simulink model "combinedfb"  (R2016a)
settings: Solver=VariableStepAuto  StartTime=0.0  StopTime=1000  RelTol=1e-3
libraries: simulink x1
settings Model: Creator=sid_1  LastModifiedBy=sid_1

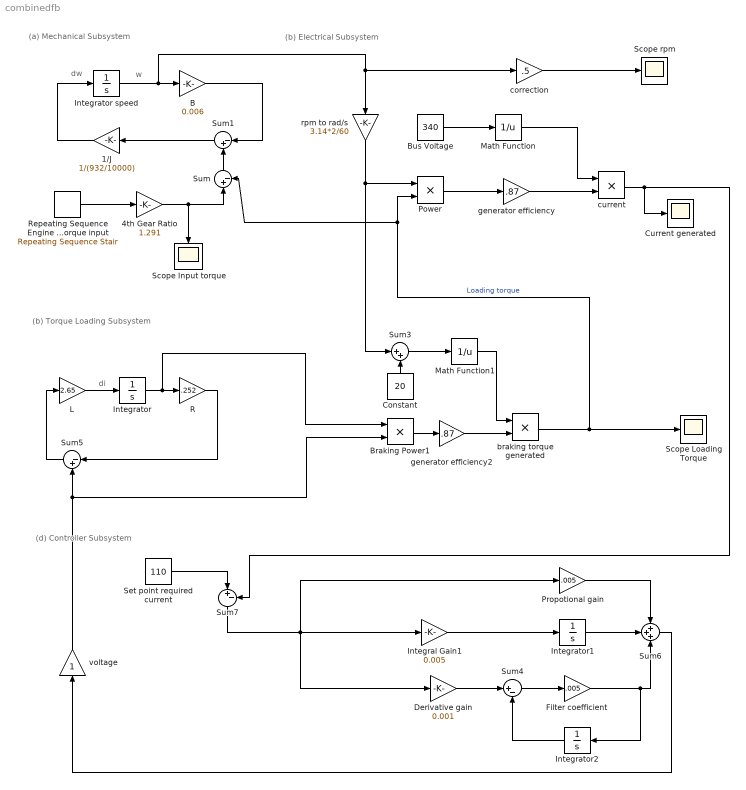
== system combinedfb ==
  note: (b) Electrical Subsystem
  note: (d) Controller Subsystem
  note: (b) Torque Loading Subsystem
  note: (a) Mechanical Subsystem
  note: dw
  note: w
  note: di
  1/J : Gain  Gain=1/(932/10000)
  4th Gear Ratio : Gain  Gain=1.291
  B : Gain  Gain=0.006
  Braking Power1 : Product
  "Bus Voltage " : Constant  Value=340
  Constant : Constant  Value=20
  Current generated : Scope
  Derivative gain : Gain  Gain=0.001
  Filter coefficient : Gain  Gain=.005
  Integral Gain1 : Gain  Gain=0.005
  Integrator : Integrator
  Integrator speed : Integrator
  Integrator1 : Integrator
  Integrator2 : Integrator
  "L " : Gain  Gain=2.65
  Math Function : Math  Operator=reciprocal  SaturateOnIntegerOverflow=on
  Math Function1 : Math  Operator=reciprocal  SaturateOnIntegerOverflow=on
  Power : Product
  Propotional gain : Gain  Gain=.005
  R : Gain  Gain=.252
  Repeating Sequence Engine Torque input : simulink/Sources/Repeating Sequence Stair  OutValues=[1:.45:77 77 77 77 77 77 77 77 77 77 77 77 77 77 77 77 77 77 77 77 77 77 77 77 77 77 77 77 77 77 77 77 77 77 77 77 77 77 77 77 77 77 77 77 77 77 77 77 77 77 77 77 77 77 77 77 77 77 77 77 77 77 77 77 77 77 77 77 77 77 77 77 77 77 77 77 77 77 77 77 77 77 77 77 77 77 77 77 77 77 77 77 77 77 77 77 77 77 77 77 77 77 77 77 77 77 77 77 77 77 77 77 77 77 77 77 77 77 77 77 77 77 77 77 77 77 77 77 77 77 77 77 77 77 77 77 77 77 77 77 77 77 77 77 77 77 77 77 77 77 77 77 77 77 77 77 77 77 77 77 77 77 77 77 77 77 77 77 77 77 77 77 77 77 77 77 77 77 77 77 77 77 77 77 77 77 77 77 77 77 77 77 77 77 77 77 77 77 77 77 77 77 77 77 77 77 77 77 77 77 77 77 77 77 77 77 77 77 77 77 77 77 77 77 77 77 77 77 77 77 77 77 77 77 77 77 77 77 77 77 77 77 77 77 77 77 77 77 77 77 77 77 77 77 77 77 77 77 77 77 77 77 77 77 77 77 77 77 77 77 77 77 77 77 77 77 77 77 77 77 77 77 77 77 77 77 77 77 77 77 77 77 77 77 77 77 77 77 77 77 77 77 77 77 77 77 77 77 77 77 77 77 77 77 77 77 77 77 77 77 77 77 77 77 77 77 77 77 77 77 77 77 77 77 77 77 77 77 77 77 77 77 77 77 77 77 77 77 77 77 77 77 77 77 77 77 77 77 77 77 77 77 77 77 77 77 77 77 77 77 77 77 77 77 77 77 77 77 77 77 77 77 77 77 77 77 77 77 77 77 77 77 77 77 77 77 77 77 77 77 77 77 77 77 77 77 77 77 77 77 77 77 77 77 77 77 77 77 77 77 77 77 77 77 77 77 77 77 77 77 77 77 77 77 77 77 77 77 77 77 77 77 77 77 77 77 77 77 77 77 77 77 77 77 77 77 77 77 77 77 77 77 77 77 77 77 77 77 77 77 77 77 77 77 77 77 77 77 77 77 77 77 77 77 77 77 77 77 77 77 77 77 77 77 77 77 77 77 77 77 77 77 77 77 77 77 77 77 77 77 77 77 77 77 77 77 77 77 77 77 77 77 77 77 77 77 77 77 77 77 77 77 77 77 77 77 77 77 77 77 77 77 77 77 77 77 77 77 77 77 77 77 77 77 77 77 77 77 77 77 77 77 77 77 77 77 77 77 77 77 77 77 77 77 77 77 77 77 77 77 77 77 77 77 77 77 77 77 77 77 77 77 77 77 77 77 77 77 77 77 77 77 77 77 77 77 77 77 77 77 77 77 77 77 77 77 77 77 77 77 77 77 77 77 77 77 77 77 77 77 77 77 77 77 77 77 77 77 77 77 77 77 77 77 77 77 77 77 77 77 77 77 77 77 77 77 77 77 77 77 77 77 77 77 77 77 77 77 77 77 77 77 77 77 77 77 77 77 77 77 77 77 77 77 77 77 77 77 77 77 77 77 77 77 77 77 77 77 77 77 77 77 77 77 77 77 77 77 77 77 77 77 77 77 77 77 77 77 77 77 77 77 77 77 77 77 77 77 77 77 77 77 77 77 77 77 77 77 77 77 77 77 77 77 77 77 77 77 77 77 77 77 77 77 77 77 77 77 77 77 77 77 77 77 77 77 77 77 77 77 77 77 77 77 77 77 77 77 77 77 77 77 77 77 77 77 77 77 77 77 77 77 77 77 77 77 77 77 77 77 77 77 77 77 77 77 77 77 77 77 77 77 77 77 77 77 77 77 77 77 77 77 77 77 77 77 77 77 77 77 77 77 77 77 77 77 77 77 77 77 77 77 77 77 77 77 77 77 77 77 77 77 77 77 77 77 77 77 77 77 77 77 77 77 77 77 77 77 77 77 77 77 77 77 77 77 77 77 77 77 77 77 77 77 77 77 77 77 77 77 77 77 77 77 77 77]  tsamp=1  OutMin=[]  OutMax=[]  OutDataTypeStr=single  OutputDataTypeScalingMode=single  OutDataType=fixdt(0,8)  ConRadixGroup=Best Precision: Vector-wise  OutScaling=2^-12
  Scope Loading Torque : Scope
  Scope rpm : Scope
  Scope Input torque : Scope
  "Set point required current " : Constant  Value=110
  Sum : Sum  Inputs=|+-
  Sum1 : Sum  Inputs=|-+
  Sum3 : Sum  Inputs=|++
  Sum4 : Sum  Inputs=|+-
  Sum5 : Sum  Inputs=|-+
  Sum6 : Sum  Inputs=+++
  Sum7 : Sum  Inputs=|+-
  braking torque generated : Product
  correction : Gain  Gain=.5
  current : Product
  generator efficiency : Gain  Gain=.87
  generator efficiency2 : Gain  Gain=.87
  rpm to rad/s : Gain  Gain=3.14*2/60
  voltage : Gain
  wires:
  Sum/1 -> Sum1/2
  Repeating Sequence Engine Torque input/1 -> 4th Gear Ratio/1
  4th Gear Ratio/1 -> Sum/1, Scope Input torque/1
  B/1 -> Sum1/1
  1/J/1 -> Integrator speed/1
  Sum1/1 -> 1/J/1
  Sum5/1 -> "L "/1
  R/1 -> Sum5/1
  generator efficiency2/1 -> braking torque generated/2
  "L "/1 -> Integrator/1
  braking torque generated/1 -> Scope Loading Torque/1, Sum/2, Power/2  "Loading torque"
  Constant/1 -> Sum3/2
  Sum3/1 -> Math Function1/1
  Braking Power1/1 -> generator efficiency2/1
  Integrator/1 -> Braking Power1/1, R/1
  Math Function1/1 -> braking torque generated/1
  voltage/1 -> Braking Power1/2, Sum5/2
  Sum6/1 -> voltage/1
  "Set point required current "/1 -> Sum7/1
  Integrator2/1 -> Sum4/2
  Integrator1/1 -> Sum6/2
  Propotional gain/1 -> Sum6/1
  Sum4/1 -> Filter coefficient/1
  Filter coefficient/1 -> Sum6/3, Integrator2/1
  Derivative gain/1 -> Sum4/1
  Integral Gain1/1 -> Integrator1/1
  Sum7/1 -> Derivative gain/1, Integral Gain1/1, Propotional gain/1
  current/1 -> Sum7/2, Current generated/1
  Integrator speed/1 -> correction/1, rpm to rad/s/1, B/1
  correction/1 -> Scope rpm/1
  generator efficiency/1 -> current/2
  Math Function/1 -> current/1
  "Bus Voltage "/1 -> Math Function/1
  Power/1 -> generator efficiency/1
  rpm to rad/s/1 -> Power/1, Sum3/1
